simulink model "FCS_MPC_6ph_Regelungsmodell"  (R2022a)
settings: Solver=ode23t  StartTime=0.0  StopTime=0.1  RelTol=1e-3  AbsTol=1e-3  EnableMultiTasking=on
values from neighbouring files (symbols this model uses):
  f_c = 100000    [Params_testbench.m]
  L_d = 0.0001473    [Params_testbench.m]
  L_q = 0.0001484    [Params_testbench.m]
  L_x = 0.00005566    (= 5.566e-05)    [Params_testbench.m]
  L_y = L_x    (= 5.566e-05)    [Params_testbench.m]
  p = 5    [Params_testbench.m]
  psi_pm = 0.0048    [Params_testbench.m]
  R_ph = 0.1278    [Params_testbench.m]
  T_100MHz = 1/f_100MHz    (= 1e-08)    [Params_testbench.m]
  u_dc = 36.0    (= 36)    [Params_testbench.m]
libraries: hdlsllib x53, nesl_utility x39, fl_lib x32, ee_lib x12, simulink x8, spsAlphaBetaZerotodq0Lib x1
(part 6 of 8)

== system FCS_MPC_6ph_Regelungsmodell/Microcontroller Software/Prediction_and_cost_function1/Subsystem ==
  d_phase_voltage_per_switching_state : Inport
  q_phase_voltage_per_switching_state : Inport  Port=2
  x_phase_voltage_per_switching_state : Inport  Port=3
  y_phase_voltage_per_switching_state : Inport  Port=4
  d_phase_voltage_per_switching_state1 : Inport  Port=5
  q_phase_voltage_per_switching_state1 : Inport  Port=6
  x_phase_voltage_per_switching_state1 : Inport  Port=7
  y_phase_voltage_per_switching_state1 : Inport  Port=8
  d_phase_voltage_per_switching_state2 : Inport  Port=9
  q_phase_voltage_per_switching_state2 : Inport  Port=10
  x_phase_voltage_per_switching_state2 : Inport  Port=11
  y_phase_voltage_per_switching_state2 : Inport  Port=12
  d_phase_voltage_per_switching_state3 : Inport  Port=13
  q_phase_voltage_per_switching_state3 : Inport  Port=14
  x_phase_voltage_per_switching_state3 : Inport  Port=15
  y_phase_voltage_per_switching_state3 : Inport  Port=16
  d_phase_voltage_per_switching_state4 : Inport  Port=17
  q_phase_voltage_per_switching_state4 : Inport  Port=18
  x_phase_voltage_per_switching_state4 : Inport  Port=19
  y_phase_voltage_per_switching_state4 : Inport  Port=20
  d_phase_voltage_per_switching_state5 : Inport  Port=21
  q_phase_voltage_per_switching_state5 : Inport  Port=22
  x_phase_voltage_per_switching_state5 : Inport  Port=23
  y_phase_voltage_per_switching_state5 : Inport  Port=24
  d_phase_voltage_per_switching_state6 : Inport  Port=25
  q_phase_voltage_per_switching_state6 : Inport  Port=26
  x_phase_voltage_per_switching_state6 : Inport  Port=27
  y_phase_voltage_per_switching_state6 : Inport  Port=28
  d_phase_voltage_per_switching_state7 : Inport  Port=29
  q_phase_voltage_per_switching_state7 : Inport  Port=30
  x_phase_voltage_per_switching_state7 : Inport  Port=31
  y_phase_voltage_per_switching_state7 : Inport  Port=32
  SampleTime_div_Ld15 : Inport  Port=33
  SampleTime_div_Lq15 : Inport  Port=34
  SampleTime_div_Lx15 : Inport  Port=35
  SampleTime_div_Ly15 : Inport  Port=36
  id_k_16 : Inport  Port=37
  iq_k_16 : Inport  Port=38
  ix_k_16 : Inport  Port=39
  iy_k_16 : Inport  Port=40
  Rs15 : Inport  Port=41
  omega_el15 : Inport  Port=42
  Lq15 : Inport  Port=43
  Ld15 : Inport  Port=44
  psiPM15 : Inport  Port=45
  id_ref15 : Inport  Port=46
  iq_ref15 : Inport  Port=47
  ix_ref15 : Inport  Port=48
  iy_ref15 : Inport  Port=49
  MATLAB Function10 : MATLAB Function  TreatAsAtomicUnit=on
  MATLAB Function11 : MATLAB Function  TreatAsAtomicUnit=on
  MATLAB Function12 : MATLAB Function  TreatAsAtomicUnit=on
  MATLAB Function13 : MATLAB Function  TreatAsAtomicUnit=on
  MATLAB Function14 : MATLAB Function  TreatAsAtomicUnit=on
  MATLAB Function15 : MATLAB Function  TreatAsAtomicUnit=on
  MATLAB Function8 : MATLAB Function  TreatAsAtomicUnit=on
  MATLAB Function9 : MATLAB Function  TreatAsAtomicUnit=on
  J : Outport
  J1 : Outport  Port=2
  J2 : Outport  Port=3
  J3 : Outport  Port=4
  J4 : Outport  Port=5
  J5 : Outport  Port=6
  J6 : Outport  Port=7
  J7 : Outport  Port=8
  wires:
  q_phase_voltage_per_switching_state1/1 -> MATLAB Function14/15(q_phase_voltage_per_switching_state)
  SampleTime_div_Ld15/1 -> MATLAB Function8/1(SampleTime_div_Ld), MATLAB Function9/1(SampleTime_div_Ld), MATLAB Function10/1(SampleTime_div_Ld), MATLAB Function11/1(SampleTime_div_Ld), MATLAB Function12/1(SampleTime_div_Ld), MATLAB Function13/1(SampleTime_div_Ld), MATLAB Function14/1(SampleTime_div_Ld), MATLAB Function15/1(SampleTime_div_Ld)
  Rs15/1 -> MATLAB Function8/9(Rs), MATLAB Function9/9(Rs), MATLAB Function10/9(Rs), MATLAB Function11/9(Rs), MATLAB Function12/9(Rs), MATLAB Function13/9(Rs), MATLAB Function14/9(Rs), MATLAB Function15/9(Rs)
  y_phase_voltage_per_switching_state/1 -> MATLAB Function15/17(y_phase_voltage_per_switching_state)
  Lq15/1 -> MATLAB Function8/11(Lq), MATLAB Function9/11(Lq), MATLAB Function10/11(Lq), MATLAB Function11/11(Lq), MATLAB Function12/11(Lq), MATLAB Function13/11(Lq), MATLAB Function14/11(Lq), MATLAB Function15/11(Lq)
  MATLAB Function11/1(J) -> J4/1
  y_phase_voltage_per_switching_state2/1 -> MATLAB Function13/17(y_phase_voltage_per_switching_state)
  d_phase_voltage_per_switching_state1/1 -> MATLAB Function14/14(d_phase_voltage_per_switching_state)
  x_phase_voltage_per_switching_state1/1 -> MATLAB Function14/16(x_phase_voltage_per_switching_state)
  y_phase_voltage_per_switching_state7/1 -> MATLAB Function8/17(y_phase_voltage_per_switching_state)
  iy_ref15/1 -> MATLAB Function8/21(iy_ref), MATLAB Function9/21(iy_ref), MATLAB Function10/21(iy_ref), MATLAB Function11/21(iy_ref), MATLAB Function12/21(iy_ref), MATLAB Function13/21(iy_ref), MATLAB Function14/21(iy_ref), MATLAB Function15/21(iy_ref)
  omega_el15/1 -> MATLAB Function8/10(omega_el), MATLAB Function9/10(omega_el), MATLAB Function10/10(omega_el), MATLAB Function11/10(omega_el), MATLAB Function12/10(omega_el), MATLAB Function13/10(omega_el), MATLAB Function14/10(omega_el), MATLAB Function15/10(omega_el)
  psiPM15/1 -> MATLAB Function8/13(psiPM), MATLAB Function9/13(psiPM), MATLAB Function10/13(psiPM), MATLAB Function11/13(psiPM), MATLAB Function12/13(psiPM), MATLAB Function13/13(psiPM), MATLAB Function14/13(psiPM), MATLAB Function15/13(psiPM)
  d_phase_voltage_per_switching_state3/1 -> MATLAB Function12/14(d_phase_voltage_per_switching_state)
  d_phase_voltage_per_switching_state6/1 -> MATLAB Function9/14(d_phase_voltage_per_switching_state)
  d_phase_voltage_per_switching_state/1 -> MATLAB Function15/14(d_phase_voltage_per_switching_state)
  x_phase_voltage_per_switching_state3/1 -> MATLAB Function12/16(x_phase_voltage_per_switching_state)
  d_phase_voltage_per_switching_state2/1 -> MATLAB Function13/14(d_phase_voltage_per_switching_state)
  x_phase_voltage_per_switching_state4/1 -> MATLAB Function11/16(x_phase_voltage_per_switching_state)
  y_phase_voltage_per_switching_state1/1 -> MATLAB Function14/17(y_phase_voltage_per_switching_state)
  MATLAB Function14/1(J) -> J1/1
  MATLAB Function8/1(J) -> J7/1
  q_phase_voltage_per_switching_state2/1 -> MATLAB Function13/15(q_phase_voltage_per_switching_state)
  x_phase_voltage_per_switching_state2/1 -> MATLAB Function13/16(x_phase_voltage_per_switching_state)
  MATLAB Function13/1(J) -> J2/1
  y_phase_voltage_per_switching_state4/1 -> MATLAB Function11/17(y_phase_voltage_per_switching_state)
  x_phase_voltage_per_switching_state/1 -> MATLAB Function15/16(x_phase_voltage_per_switching_state)
  q_phase_voltage_per_switching_state5/1 -> MATLAB Function10/15(q_phase_voltage_per_switching_state)
  d_phase_voltage_per_switching_state7/1 -> MATLAB Function8/14(d_phase_voltage_per_switching_state)
  d_phase_voltage_per_switching_state4/1 -> MATLAB Function11/14(d_phase_voltage_per_switching_state)
  q_phase_voltage_per_switching_state4/1 -> MATLAB Function11/15(q_phase_voltage_per_switching_state)
  x_phase_voltage_per_switching_state5/1 -> MATLAB Function10/16(x_phase_voltage_per_switching_state)
  SampleTime_div_Lx15/1 -> MATLAB Function8/3(SampleTime_div_Lx), MATLAB Function9/3(SampleTime_div_Lx), MATLAB Function10/3(SampleTime_div_Lx), MATLAB Function11/3(SampleTime_div_Lx), MATLAB Function12/3(SampleTime_div_Lx), MATLAB Function13/3(SampleTime_div_Lx), MATLAB Function14/3(SampleTime_div_Lx), MATLAB Function15/3(SampleTime_div_Lx)
  SampleTime_div_Ly15/1 -> MATLAB Function8/4(SampleTime_div_Ly), MATLAB Function9/4(SampleTime_div_Ly), MATLAB Function10/4(SampleTime_div_Ly), MATLAB Function11/4(SampleTime_div_Ly), MATLAB Function12/4(SampleTime_div_Ly), MATLAB Function13/4(SampleTime_div_Ly), MATLAB Function14/4(SampleTime_div_Ly), MATLAB Function15/4(SampleTime_div_Ly)
  SampleTime_div_Lq15/1 -> MATLAB Function8/2(SampleTime_div_Lq), MATLAB Function9/2(SampleTime_div_Lq), MATLAB Function10/2(SampleTime_div_Lq), MATLAB Function11/2(SampleTime_div_Lq), MATLAB Function12/2(SampleTime_div_Lq), MATLAB Function13/2(SampleTime_div_Lq), MATLAB Function14/2(SampleTime_div_Lq), MATLAB Function15/2(SampleTime_div_Lq)
  x_phase_voltage_per_switching_state7/1 -> MATLAB Function8/16(x_phase_voltage_per_switching_state)
  q_phase_voltage_per_switching_state/1 -> MATLAB Function15/15(q_phase_voltage_per_switching_state)
  MATLAB Function15/1(J) -> J/1
  d_phase_voltage_per_switching_state5/1 -> MATLAB Function10/14(d_phase_voltage_per_switching_state)
  MATLAB Function10/1(J) -> J5/1
  y_phase_voltage_per_switching_state5/1 -> MATLAB Function10/17(y_phase_voltage_per_switching_state)
  q_phase_voltage_per_switching_state6/1 -> MATLAB Function9/15(q_phase_voltage_per_switching_state)
  y_phase_voltage_per_switching_state6/1 -> MATLAB Function9/17(y_phase_voltage_per_switching_state)
  x_phase_voltage_per_switching_state6/1 -> MATLAB Function9/16(x_phase_voltage_per_switching_state)
  MATLAB Function9/1(J) -> J6/1
  MATLAB Function12/1(J) -> J3/1
  q_phase_voltage_per_switching_state7/1 -> MATLAB Function8/15(q_phase_voltage_per_switching_state)
  y_phase_voltage_per_switching_state3/1 -> MATLAB Function12/17(y_phase_voltage_per_switching_state)
  q_phase_voltage_per_switching_state3/1 -> MATLAB Function12/15(q_phase_voltage_per_switching_state)
  ix_ref15/1 -> MATLAB Function8/20(ix_ref), MATLAB Function9/20(ix_ref), MATLAB Function10/20(ix_ref), MATLAB Function11/20(ix_ref), MATLAB Function12/20(ix_ref), MATLAB Function13/20(ix_ref), MATLAB Function14/20(ix_ref), MATLAB Function15/20(ix_ref)
  iq_ref15/1 -> MATLAB Function8/19(iq_ref), MATLAB Function9/19(iq_ref), MATLAB Function10/19(iq_ref), MATLAB Function11/19(iq_ref), MATLAB Function12/19(iq_ref), MATLAB Function13/19(iq_ref), MATLAB Function14/19(iq_ref), MATLAB Function15/19(iq_ref)
  id_ref15/1 -> MATLAB Function8/18(id_ref), MATLAB Function9/18(id_ref), MATLAB Function10/18(id_ref), MATLAB Function11/18(id_ref), MATLAB Function12/18(id_ref), MATLAB Function13/18(id_ref), MATLAB Function14/18(id_ref), MATLAB Function15/18(id_ref)
  Ld15/1 -> MATLAB Function8/12(Ld), MATLAB Function9/12(Ld), MATLAB Function10/12(Ld), MATLAB Function11/12(Ld), MATLAB Function12/12(Ld), MATLAB Function13/12(Ld), MATLAB Function14/12(Ld), MATLAB Function15/12(Ld)
  iy_k_16/1 -> MATLAB Function8/8(iy_k_1), MATLAB Function9/8(iy_k_1), MATLAB Function10/8(iy_k_1), MATLAB Function11/8(iy_k_1), MATLAB Function12/8(iy_k_1), MATLAB Function13/8(iy_k_1), MATLAB Function14/8(iy_k_1), MATLAB Function15/8(iy_k_1)
  ix_k_16/1 -> MATLAB Function8/7(ix_k_1), MATLAB Function9/7(ix_k_1), MATLAB Function10/7(ix_k_1), MATLAB Function11/7(ix_k_1), MATLAB Function12/7(ix_k_1), MATLAB Function13/7(ix_k_1), MATLAB Function14/7(ix_k_1), MATLAB Function15/7(ix_k_1)
  iq_k_16/1 -> MATLAB Function8/6(iq_k_1), MATLAB Function9/6(iq_k_1), MATLAB Function10/6(iq_k_1), MATLAB Function11/6(iq_k_1), MATLAB Function12/6(iq_k_1), MATLAB Function13/6(iq_k_1), MATLAB Function14/6(iq_k_1), MATLAB Function15/6(iq_k_1)
  id_k_16/1 -> MATLAB Function8/5(id_k_1), MATLAB Function9/5(id_k_1), MATLAB Function10/5(id_k_1), MATLAB Function11/5(id_k_1), MATLAB Function12/5(id_k_1), MATLAB Function13/5(id_k_1), MATLAB Function14/5(id_k_1), MATLAB Function15/5(id_k_1)

== matlab function FCS_MPC_6ph_Regelungsmodell/Microcontroller Software/Phase_voltages_per_switching_state2/MATLAB Function1 ==
  settings: fimath=fimath('RoundingMethod', 'Floor','OverflowAction', 'Wrap','ProductMode', 'FullPrecision', 'SumMode', 'FullPrecision')
  data: u input; y output
function y = fcn(u)

    y = fi(u*(1/(2*pi)));

end

== matlab function FCS_MPC_6ph_Regelungsmodell/Microcontroller Software/vsd_and_park_tra1/MATLAB Function ==
  settings: fimath=fimath('RoundingMethod', 'Floor','OverflowAction', 'Wrap','ProductMode', 'FullPrecision', 'SumMode', 'FullPrecision')
  data: i_a1 input; i_alpha output; i_b1 input; i_c1 input; i_a2 input; i_b2 input; i_c2 input; sin_theta_el input; i_beta output; i_x output; i_y output; i_0_plus output; i_0_minus output; i_d output; i_q output; cos_theta_el input
function [i_alpha,i_beta,i_x,i_y,i_0_plus,i_0_minus,i_d,i_q] = VSD_and_Park_transformation(i_a1,i_b1,i_c1,i_a2,i_b2,i_c2,sin_theta_el,cos_theta_el)

    % VSD-Transformation
    A = [0 0 0 0 0 0]';

    A =  0.3333*[1    -0.5        -0.5        0.8660   -0.8660  0 ;
                0    0.8660   -0.8660  0.5         0.5         -1;
                1    -0.5        -0.5        -0.8660  0.8660   0 ;
                0    -0.8660  0.8660   0.5         0.5         -1;
                1    1           1           0           0           0 ;
                0    0           0           1           1           1] * [i_a1 i_b1 i_c1 i_a2 i_b2 i_c2]';

    i_alpha = A(1);
    i_beta = A(2);
    i_x = A(3);
    i_y = A(4);
    i_0_plus = A(5);
    i_0_minus = A(6);

    % Park-Transformation
%    B = [0 0]';

%     B = [cos(theta_el)       sin(theta_el);
%         -sin(theta_el)       cos(theta_el)] * [i_alpha i_beta]';

 %   i_d = B(1);
 %   i_q = B(2);



i_d = cos_theta_el*i_alpha+sin_theta_el*i_beta;
i_q = -sin_theta_el*i_alpha+cos_theta_el*i_beta;


end

== matlab function FCS_MPC_6ph_Regelungsmodell/Microcontroller Software/vsd_and_park_tra1/MATLAB Function1 ==
  settings: fimath=fimath('RoundingMethod', 'Floor','OverflowAction', 'Wrap','ProductMode', 'FullPrecision', 'SumMode', 'FullPrecision')
  data: u input; y output
function y = fcn(u)

    y = u*(1/(2*pi));

end

== matlab function FCS_MPC_6ph_Regelungsmodell/Microcontroller Software/Delay_compensation1/MATLAB Function ==
  data: SampleTime_div_Ld input; SampleTime_div_Lq input; SampleTime_div_Lx input; SampleTime_div_Ly input; id_k_1 output; last_applied_optimal_voltage_d input; last_applied_optimal_voltage_q input; last_applied_optimal_voltage_x input; last_applied_optimal_voltage_y input; id_measured input; iq_measured input; ix_measured input; iy_measured input; psiPM input; Lq input; Ld input; Rs input; iq_k_1 output; ix_k_1 output; iy_k_1 output; omega_el input
function [id_k_1, iq_k_1, ix_k_1, iy_k_1] = fcn(SampleTime_div_Ld, SampleTime_div_Lq, SampleTime_div_Lx, SampleTime_div_Ly, last_applied_optimal_voltage_d, last_applied_optimal_voltage_q, last_applied_optimal_voltage_x, last_applied_optimal_voltage_y, id_measured, iq_measured, ix_measured, iy_measured, psiPM, Lq, Ld, Rs, omega_el)
  
    % Delay compensation with a modell of a 6-Phase PMSM
    id_k_1 = single(SampleTime_div_Ld*(last_applied_optimal_voltage_d-id_measured*Rs+omega_el*Lq*iq_measured)+id_measured);
    iq_k_1 = single(SampleTime_div_Lq*(last_applied_optimal_voltage_q-iq_measured*Rs-omega_el*(psiPM+id_measured*Ld))+iq_measured);
    ix_k_1 = single(SampleTime_div_Lx*(last_applied_optimal_voltage_x-ix_measured*Rs)+ix_measured);
    iy_k_1 = single(SampleTime_div_Ly*(last_applied_optimal_voltage_y-iy_measured*Rs)+iy_measured);

end

== matlab function FCS_MPC_6ph_Regelungsmodell/Microcontroller Software/Prediction_and_cost_function1/Subsystem/MATLAB Function10 ==
  data: SampleTime_div_Ld input; J output; SampleTime_div_Lq input; SampleTime_div_Lx input; SampleTime_div_Ly input; id_k_1 input; iq_k_1 input; ix_k_1 input; iy_k_1 input; Rs input; omega_el input; Lq input; Ld input; psiPM input; d_phase_voltage_per_switching_state input; q_phase_voltage_per_switching_state input; x_phase_voltage_per_switching_state input; y_phase_voltage_per_switching_state input; id_ref input; iq_ref input; ix_ref input; iy_ref input
function J = fcn(SampleTime_div_Ld, SampleTime_div_Lq, SampleTime_div_Lx, SampleTime_div_Ly, id_k_1, iq_k_1, ix_k_1, iy_k_1, Rs, omega_el, Lq, Ld, psiPM, d_phase_voltage_per_switching_state, q_phase_voltage_per_switching_state, x_phase_voltage_per_switching_state, y_phase_voltage_per_switching_state, id_ref, iq_ref, ix_ref, iy_ref)
     
        % Prediction of the d-, q-, x-, y-currents of the 6-Phase-PMSM with the finite control set 
        id_k_2 = single(SampleTime_div_Ld*(d_phase_voltage_per_switching_state-id_k_1*Rs+omega_el*Lq*iq_k_1)+id_k_1);
        iq_k_2 = single(SampleTime_div_Lq*(q_phase_voltage_per_switching_state-iq_k_1*Rs-omega_el*(psiPM+id_k_1*Ld))+iq_k_1);
        ix_k_2 = single(SampleTime_div_Lx*(x_phase_voltage_per_switching_state-ix_k_1*Rs)+ix_k_1);
        iy_k_2 = single(SampleTime_div_Ly*(y_phase_voltage_per_switching_state-iy_k_1*Rs)+iy_k_1);
        
        % Calculation of the cost function
        J = single((id_ref-id_k_2)^2+(iq_ref-iq_k_2)^2+(ix_ref-ix_k_2)^2+(iy_ref-iy_k_2)^2);

end

== matlab function FCS_MPC_6ph_Regelungsmodell/Microcontroller Software/Prediction_and_cost_function1/Subsystem/MATLAB Function11 ==
  data: SampleTime_div_Ld input; J output; SampleTime_div_Lq input; SampleTime_div_Lx input; SampleTime_div_Ly input; id_k_1 input; iq_k_1 input; ix_k_1 input; iy_k_1 input; Rs input; omega_el input; Lq input; Ld input; psiPM input; d_phase_voltage_per_switching_state input; q_phase_voltage_per_switching_state input; x_phase_voltage_per_switching_state input; y_phase_voltage_per_switching_state input; id_ref input; iq_ref input; ix_ref input; iy_ref input
function J = fcn(SampleTime_div_Ld, SampleTime_div_Lq, SampleTime_div_Lx, SampleTime_div_Ly, id_k_1, iq_k_1, ix_k_1, iy_k_1, Rs, omega_el, Lq, Ld, psiPM, d_phase_voltage_per_switching_state, q_phase_voltage_per_switching_state, x_phase_voltage_per_switching_state, y_phase_voltage_per_switching_state, id_ref, iq_ref, ix_ref, iy_ref)
     
        % Prediction of the d-, q-, x-, y-currents of the 6-Phase-PMSM with the finite control set 
        id_k_2 = single(SampleTime_div_Ld*(d_phase_voltage_per_switching_state-id_k_1*Rs+omega_el*Lq*iq_k_1)+id_k_1);
        iq_k_2 = single(SampleTime_div_Lq*(q_phase_voltage_per_switching_state-iq_k_1*Rs-omega_el*(psiPM+id_k_1*Ld))+iq_k_1);
        ix_k_2 = single(SampleTime_div_Lx*(x_phase_voltage_per_switching_state-ix_k_1*Rs)+ix_k_1);
        iy_k_2 = single(SampleTime_div_Ly*(y_phase_voltage_per_switching_state-iy_k_1*Rs)+iy_k_1);
        
        % Calculation of the cost function
        J = single((id_ref-id_k_2)^2+(iq_ref-iq_k_2)^2+(ix_ref-ix_k_2)^2+(iy_ref-iy_k_2)^2);

end

== matlab function FCS_MPC_6ph_Regelungsmodell/Microcontroller Software/Prediction_and_cost_function1/Subsystem/MATLAB Function12 ==
  data: SampleTime_div_Ld input; J output; SampleTime_div_Lq input; SampleTime_div_Lx input; SampleTime_div_Ly input; id_k_1 input; iq_k_1 input; ix_k_1 input; iy_k_1 input; Rs input; omega_el input; Lq input; Ld input; psiPM input; d_phase_voltage_per_switching_state input; q_phase_voltage_per_switching_state input; x_phase_voltage_per_switching_state input; y_phase_voltage_per_switching_state input; id_ref input; iq_ref input; ix_ref input; iy_ref input
function J = fcn(SampleTime_div_Ld, SampleTime_div_Lq, SampleTime_div_Lx, SampleTime_div_Ly, id_k_1, iq_k_1, ix_k_1, iy_k_1, Rs, omega_el, Lq, Ld, psiPM, d_phase_voltage_per_switching_state, q_phase_voltage_per_switching_state, x_phase_voltage_per_switching_state, y_phase_voltage_per_switching_state, id_ref, iq_ref, ix_ref, iy_ref)
     
        % Prediction of the d-, q-, x-, y-currents of the 6-Phase-PMSM with the finite control set 
        id_k_2 = single(SampleTime_div_Ld*(d_phase_voltage_per_switching_state-id_k_1*Rs+omega_el*Lq*iq_k_1)+id_k_1);
        iq_k_2 = single(SampleTime_div_Lq*(q_phase_voltage_per_switching_state-iq_k_1*Rs-omega_el*(psiPM+id_k_1*Ld))+iq_k_1);
        ix_k_2 = single(SampleTime_div_Lx*(x_phase_voltage_per_switching_state-ix_k_1*Rs)+ix_k_1);
        iy_k_2 = single(SampleTime_div_Ly*(y_phase_voltage_per_switching_state-iy_k_1*Rs)+iy_k_1);
        
        % Calculation of the cost function
        J = single((id_ref-id_k_2)^2+(iq_ref-iq_k_2)^2+(ix_ref-ix_k_2)^2+(iy_ref-iy_k_2)^2);

end

== matlab function FCS_MPC_6ph_Regelungsmodell/Microcontroller Software/Prediction_and_cost_function1/Subsystem/MATLAB Function13 ==
  data: SampleTime_div_Ld input; J output; SampleTime_div_Lq input; SampleTime_div_Lx input; SampleTime_div_Ly input; id_k_1 input; iq_k_1 input; ix_k_1 input; iy_k_1 input; Rs input; omega_el input; Lq input; Ld input; psiPM input; d_phase_voltage_per_switching_state input; q_phase_voltage_per_switching_state input; x_phase_voltage_per_switching_state input; y_phase_voltage_per_switching_state input; id_ref input; iq_ref input; ix_ref input; iy_ref input
function J = fcn(SampleTime_div_Ld, SampleTime_div_Lq, SampleTime_div_Lx, SampleTime_div_Ly, id_k_1, iq_k_1, ix_k_1, iy_k_1, Rs, omega_el, Lq, Ld, psiPM, d_phase_voltage_per_switching_state, q_phase_voltage_per_switching_state, x_phase_voltage_per_switching_state, y_phase_voltage_per_switching_state, id_ref, iq_ref, ix_ref, iy_ref)
     
        % Prediction of the d-, q-, x-, y-currents of the 6-Phase-PMSM with the finite control set 
        id_k_2 = single(SampleTime_div_Ld*(d_phase_voltage_per_switching_state-id_k_1*Rs+omega_el*Lq*iq_k_1)+id_k_1);
        iq_k_2 = single(SampleTime_div_Lq*(q_phase_voltage_per_switching_state-iq_k_1*Rs-omega_el*(psiPM+id_k_1*Ld))+iq_k_1);
        ix_k_2 = single(SampleTime_div_Lx*(x_phase_voltage_per_switching_state-ix_k_1*Rs)+ix_k_1);
        iy_k_2 = single(SampleTime_div_Ly*(y_phase_voltage_per_switching_state-iy_k_1*Rs)+iy_k_1);
        
        % Calculation of the cost function
        J = single((id_ref-id_k_2)^2+(iq_ref-iq_k_2)^2+(ix_ref-ix_k_2)^2+(iy_ref-iy_k_2)^2);

end

== matlab function FCS_MPC_6ph_Regelungsmodell/Microcontroller Software/Switching_states/MATLAB Function1 ==
  data: I input; next_switching_state output
function next_switching_state = fcn(I)

    % Possible switching states of the 6-Phase 2-level inverter
    possible_swichting_states = [0	1	0	1	0	1	0	1	0	1	0	1;
                                1	0	0	1	0	1	0	1	0	1	0	1;
                                0	1	1	0	0	1	0	1	0	1	0	1;
                                1	0	1	0	0	1	0	1	0	1	0	1;
                                0	1	0	1	1	0	0	1	0	1	0	1;
                                1	0	0	1	1	0	0	1	0	1	0	1;
                                0	1	1	0	1	0	0	1	0	1	0	1;
                                1	0	1	0	1	0	0	1	0	1	0	1;
                                0	1	0	1	0	1	1	0	0	1	0	1;
                                1	0	0	1	0	1	1	0	0	1	0	1;
                                0	1	1	0	0	1	1	0	0	1	0	1;
                                1	0	1	0	0	1	1	0	0	1	0	1;
                                0	1	0	1	1	0	1	0	0	1	0	1;
                                1	0	0	1	1	0	1	0	0	1	0	1;
                                0	1	1	0	1	0	1	0	0	1	0	1;
                                1	0	1	0	1	0	1	0	0	1	0	1;
                                0	1	0	1	0	1	0	1	1	0	0	1;
                                1	0	0	1	0	1	0	1	1	0	0	1;
                                0	1	1	0	0	1	0	1	1	0	0	1;
                                1	0	1	0	0	1	0	1	1	0	0	1;
                                0	1	0	1	1	0	0	1	1	0	0	1;
                                1	0	0	1	1	0	0	1	1	0	0	1;
                                0	1	1	0	1	0	0	1	1	0	0	1;
                                1	0	1	0	1	0	0	1	1	0	0	1;
                                0	1	0	1	0	1	1	0	1	0	0	1;
                                1	0	0	1	0	1	1	0	1	0	0	1;
                                0	1	1	0	0	1	1	0	1	0	0	1;
                                1	0	1	0	0	1	1	0	1	0	0	1;
                                0	1	0	1	1	0	1	0	1	0	0	1;
                                1	0	0	1	1	0	1	0	1	0	0	1;
                                0	1	1	0	1	0	1	0	1	0	0	1;
                                1	0	1	0	1	0	1	0	1	0	0	1;
                                0	1	0	1	0	1	0	1	0	1	1	0;
                                1	0	0	1	0	1	0	1	0	1	1	0;
                                0	1	1	0	0	1	0	1	0	1	1	0;
                                1	0	1	0	0	1	0	1	0	1	1	0;
                                0	1	0	1	1	0	0	1	0	1	1	0;
                                1	0	0	1	1	0	0	1	0	1	1	0;
                                0	1	1	0	1	0	0	1	0	1	1	0;
                                1	0	1	0	1	0	0	1	0	1	1	0;
                                0	1	0	1	0	1	1	0	0	1	1	0;
                                1	0	0	1	0	1	1	0	0	1	1	0;
                                0	1	1	0	0	1	1	0	0	1	1	0;
                                1	0	1	0	0	1	1	0	0	1	1	0;
                                0	1	0	1	1	0	1	0	0	1	1	0;
                                1	0	0	1	1	0	1	0	0	1	1	0;
                                0	1	1	0	1	0	1	0	0	1	1	0;
                                1	0	1	0	1	0	1	0	0	1	1	0;
                                0	1	0	1	0	1	0	1	1	0	1	0;
                                1	0	0	1	0	1	0	1	1	0	1	0;
                                0	1	1	0	0	1	0	1	1	0	1	0;
                                1	0	1	0	0	1	0	1	1	0	1	0;
                                0	1	0	1	1	0	0	1	1	0	1	0;
                                1	0	0	1	1	0	0	1	1	0	1	0;
                                0	1	1	0	1	0	0	1	1	0	1	0;
                                1	0	1	0	1	0	0	1	1	0	1	0;
                                0	1	0	1	0	1	1	0	1	0	1	0;
                                1	0	0	1	0	1	1	0	1	0	1	0;
                                0	1	1	0	0	1	1	0	1	0	1	0;
                                1	0	1	0	0	1	1	0	1	0	1	0;
                                0	1	0	1	1	0	1	0	1	0	1	0;
                                1	0	0	1	1	0	1	0	1	0	1	0;
                                0	1	1	0	1	0	1	0	1	0	1	0;
                                1	0	1	0	1	0	1	0	1	0	1	0];

    % Initial condition
    if I==0
        I=int32(1);
    end

    % Output switching state
    next_switching_state=boolean(possible_swichting_states(I,:))';

end

== matlab function FCS_MPC_6ph_Regelungsmodell/6ph_PMSM_30deg_VSD1 ==
  data: u1 input; y1 output; u2 input; u3 input; u4 input; u5 input; u6 input; y2 output; y3 output; y4 output; y5 output; y6 output; k6 input; c6 input
function [y1,y2,y3,y4,y5,y6] = VSD_asymm_30(u1,u2,u3,u4,u5,u6,k6,c6)

A =single([0 0 0 0 0 0]');

A =    k6*[1    -0.5        -0.5        sqrt(3)/2   -sqrt(3)/2  0 ;
           0    sqrt(3)/2   -sqrt(3)/2  0.5         0.5         -1;
           1    -0.5        -0.5        -sqrt(3)/2  sqrt(3)/2   0 ;
           0    -sqrt(3)/2  sqrt(3)/2   0.5         0.5         -1;
           c6   c6          c6          0           0           0 ;
           0    0           0           c6          c6          c6] * [u1 u2 u3 u4 u5 u6]';

y1 =single(A(1));
y2 =single(A(2));
y3 =single(A(3));
y4 =single(A(4));
y5 =single(A(5));
y6 =single(A(6));

== matlab function FCS_MPC_6ph_Regelungsmodell/Microcontroller Software/Prediction_and_cost_function1/Subsystem/MATLAB Function14 ==
  data: SampleTime_div_Ld input; J output; SampleTime_div_Lq input; SampleTime_div_Lx input; SampleTime_div_Ly input; id_k_1 input; iq_k_1 input; ix_k_1 input; iy_k_1 input; Rs input; omega_el input; Lq input; Ld input; psiPM input; d_phase_voltage_per_switching_state input; q_phase_voltage_per_switching_state input; x_phase_voltage_per_switching_state input; y_phase_voltage_per_switching_state input; id_ref input; iq_ref input; ix_ref input; iy_ref input
function J = fcn(SampleTime_div_Ld, SampleTime_div_Lq, SampleTime_div_Lx, SampleTime_div_Ly, id_k_1, iq_k_1, ix_k_1, iy_k_1, Rs, omega_el, Lq, Ld, psiPM, d_phase_voltage_per_switching_state, q_phase_voltage_per_switching_state, x_phase_voltage_per_switching_state, y_phase_voltage_per_switching_state, id_ref, iq_ref, ix_ref, iy_ref)
     
        % Prediction of the d-, q-, x-, y-currents of the 6-Phase-PMSM with the finite control set 
        id_k_2 = single(SampleTime_div_Ld*(d_phase_voltage_per_switching_state-id_k_1*Rs+omega_el*Lq*iq_k_1)+id_k_1);
        iq_k_2 = single(SampleTime_div_Lq*(q_phase_voltage_per_switching_state-iq_k_1*Rs-omega_el*(psiPM+id_k_1*Ld))+iq_k_1);
        ix_k_2 = single(SampleTime_div_Lx*(x_phase_voltage_per_switching_state-ix_k_1*Rs)+ix_k_1);
        iy_k_2 = single(SampleTime_div_Ly*(y_phase_voltage_per_switching_state-iy_k_1*Rs)+iy_k_1);
        
        % Calculation of the cost function
        J = single((id_ref-id_k_2)^2+(iq_ref-iq_k_2)^2+(ix_ref-ix_k_2)^2+(iy_ref-iy_k_2)^2);

end

== matlab function FCS_MPC_6ph_Regelungsmodell/Microcontroller Software/Prediction_and_cost_function1/Subsystem/MATLAB Function15 ==
  data: SampleTime_div_Ld input; J output; SampleTime_div_Lq input; SampleTime_div_Lx input; SampleTime_div_Ly input; id_k_1 input; iq_k_1 input; ix_k_1 input; iy_k_1 input; Rs input; omega_el input; Lq input; Ld input; psiPM input; d_phase_voltage_per_switching_state input; q_phase_voltage_per_switching_state input; x_phase_voltage_per_switching_state input; y_phase_voltage_per_switching_state input; id_ref input; iq_ref input; ix_ref input; iy_ref input
function J = fcn(SampleTime_div_Ld, SampleTime_div_Lq, SampleTime_div_Lx, SampleTime_div_Ly, id_k_1, iq_k_1, ix_k_1, iy_k_1, Rs, omega_el, Lq, Ld, psiPM, d_phase_voltage_per_switching_state, q_phase_voltage_per_switching_state, x_phase_voltage_per_switching_state, y_phase_voltage_per_switching_state, id_ref, iq_ref, ix_ref, iy_ref)
     
        % Prediction of the d-, q-, x-, y-currents of the 6-Phase-PMSM with the finite control set 
        id_k_2 = single(SampleTime_div_Ld*(d_phase_voltage_per_switching_state-id_k_1*Rs+omega_el*Lq*iq_k_1)+id_k_1);
        iq_k_2 = single(SampleTime_div_Lq*(q_phase_voltage_per_switching_state-iq_k_1*Rs-omega_el*(psiPM+id_k_1*Ld))+iq_k_1);
        ix_k_2 = single(SampleTime_div_Lx*(x_phase_voltage_per_switching_state-ix_k_1*Rs)+ix_k_1);
        iy_k_2 = single(SampleTime_div_Ly*(y_phase_voltage_per_switching_state-iy_k_1*Rs)+iy_k_1);
        
        % Calculation of the cost function
        J = single((id_ref-id_k_2)^2+(iq_ref-iq_k_2)^2+(ix_ref-ix_k_2)^2+(iy_ref-iy_k_2)^2);

end

== matlab function FCS_MPC_6ph_Regelungsmodell/Microcontroller Software/Prediction_and_cost_function1/Subsystem/MATLAB Function8 ==
  data: SampleTime_div_Ld input; J output; SampleTime_div_Lq input; SampleTime_div_Lx input; SampleTime_div_Ly input; id_k_1 input; iq_k_1 input; ix_k_1 input; iy_k_1 input; Rs input; omega_el input; Lq input; Ld input; psiPM input; d_phase_voltage_per_switching_state input; q_phase_voltage_per_switching_state input; x_phase_voltage_per_switching_state input; y_phase_voltage_per_switching_state input; id_ref input; iq_ref input; ix_ref input; iy_ref input
function J = fcn(SampleTime_div_Ld, SampleTime_div_Lq, SampleTime_div_Lx, SampleTime_div_Ly, id_k_1, iq_k_1, ix_k_1, iy_k_1, Rs, omega_el, Lq, Ld, psiPM, d_phase_voltage_per_switching_state, q_phase_voltage_per_switching_state, x_phase_voltage_per_switching_state, y_phase_voltage_per_switching_state, id_ref, iq_ref, ix_ref, iy_ref)
     
        % Prediction of the d-, q-, x-, y-currents of the 6-Phase-PMSM with the finite control set 
        id_k_2 = single(SampleTime_div_Ld*(d_phase_voltage_per_switching_state-id_k_1*Rs+omega_el*Lq*iq_k_1)+id_k_1);
        iq_k_2 = single(SampleTime_div_Lq*(q_phase_voltage_per_switching_state-iq_k_1*Rs-omega_el*(psiPM+id_k_1*Ld))+iq_k_1);
        ix_k_2 = single(SampleTime_div_Lx*(x_phase_voltage_per_switching_state-ix_k_1*Rs)+ix_k_1);
        iy_k_2 = single(SampleTime_div_Ly*(y_phase_voltage_per_switching_state-iy_k_1*Rs)+iy_k_1);
        
        % Calculation of the cost function
        J = single((id_ref-id_k_2)^2+(iq_ref-iq_k_2)^2+(ix_ref-ix_k_2)^2+(iy_ref-iy_k_2)^2);

end

== matlab function FCS_MPC_6ph_Regelungsmodell/Microcontroller Software/Prediction_and_cost_function1/Subsystem/MATLAB Function9 ==
  data: SampleTime_div_Ld input; J output; SampleTime_div_Lq input; SampleTime_div_Lx input; SampleTime_div_Ly input; id_k_1 input; iq_k_1 input; ix_k_1 input; iy_k_1 input; Rs input; omega_el input; Lq input; Ld input; psiPM input; d_phase_voltage_per_switching_state input; q_phase_voltage_per_switching_state input; x_phase_voltage_per_switching_state input; y_phase_voltage_per_switching_state input; id_ref input; iq_ref input; ix_ref input; iy_ref input
function J = fcn(SampleTime_div_Ld, SampleTime_div_Lq, SampleTime_div_Lx, SampleTime_div_Ly, id_k_1, iq_k_1, ix_k_1, iy_k_1, Rs, omega_el, Lq, Ld, psiPM, d_phase_voltage_per_switching_state, q_phase_voltage_per_switching_state, x_phase_voltage_per_switching_state, y_phase_voltage_per_switching_state, id_ref, iq_ref, ix_ref, iy_ref)
     
        % Prediction of the d-, q-, x-, y-currents of the 6-Phase-PMSM with the finite control set 
        id_k_2 = single(SampleTime_div_Ld*(d_phase_voltage_per_switching_state-id_k_1*Rs+omega_el*Lq*iq_k_1)+id_k_1);
        iq_k_2 = single(SampleTime_div_Lq*(q_phase_voltage_per_switching_state-iq_k_1*Rs-omega_el*(psiPM+id_k_1*Ld))+iq_k_1);
        ix_k_2 = single(SampleTime_div_Lx*(x_phase_voltage_per_switching_state-ix_k_1*Rs)+ix_k_1);
        iy_k_2 = single(SampleTime_div_Ly*(y_phase_voltage_per_switching_state-iy_k_1*Rs)+iy_k_1);
        
        % Calculation of the cost function
        J = single((id_ref-id_k_2)^2+(iq_ref-iq_k_2)^2+(ix_ref-ix_k_2)^2+(iy_ref-iy_k_2)^2);

end

== matlab function FCS_MPC_6ph_Regelungsmodell/Microcontroller Software/Min_cost_function_and_vopt1/MATLAB Function ==
  data: J_1 input fixdt(1,20,11); Index_1 input int32; J output fixdt(1,20,11); voltages_1 input fixdt(1,24,11); J_2 input fixdt(1,20,11); Index_2 input int32; voltages_2 input fixdt(1,24,11); J_3 input fixdt(1,20,11); Index_3 input int32; voltages_3 input fixdt(1,24,11); J_4 input fixdt(1,20,11); Index_4 input int32; voltages_4 input fixdt(1,24,11); J_5 input fixdt(1,20,11); Index_5 input int32; voltages_5 input fixdt(1,24,11); J_6 input fixdt(1,20,11); Index_6 input; voltages_6 input fixdt(1,24,11); J_7 input fixdt(1,20,11); Index_7 input int32; voltages_7 input fixdt(1,24,11); J_8 input fixdt(1,20,11); Index_8 input int32; voltages_8 input fixdt(1,24,11); Index output int32; voltages output fixdt(1,24,11); min input fixdt(1,20,11); J_default input fixdt(1,20,11); voltages_default input fixdt(1,24,11)
function [J, Index, voltages] = fcn(J_1, Index_1, voltages_1, J_2, Index_2, voltages_2, J_3, Index_3, voltages_3, J_4, Index_4, voltages_4, J_5, Index_5, voltages_5, J_6, Index_6, voltages_6, ...
                                    J_7, Index_7, voltages_7, J_8, Index_8, voltages_8, min, J_default,voltages_default)



if J_1 == min
    Index = Index_1;
    voltages = voltages_1;
    J = J_1;
elseif J_2 == min
    Index = Index_2;
    voltages = voltages_2;
    J = J_2;
elseif J_3 == min
    Index = Index_3;
    voltages = voltages_3;
    J = J_3;
elseif J_4 == min
    Index = Index_4;
    voltages = voltages_4;
    J = J_4;
elseif J_5 == min
    Index = Index_5;
    voltages = voltages_5;
    J = J_5;
elseif J_6 == min
    Index = Index_6;
    voltages = voltages_6;
    J = J_6;
elseif J_7 == min
    Index = Index_7;
    voltages = voltages_7;
    J = J_7;
elseif J_8 == min
    Index = Index_8;
    voltages = voltages_8;
    J = J_8;
else 
    Index = int32(0);
    J = J_default;
    voltages = voltages_default;
end

== matlab function FCS_MPC_6ph_Regelungsmodell/Microcontroller Software/Switching_states1/MATLAB Function1 ==
  data: I input; next_switching_state output
function next_switching_state = fcn(I)

    % Possible switching states of the 6-Phase 2-level inverter
    possible_swichting_states = [0	1	0	1	0	1	0	1	0	1	0	1;
                                1	0	0	1	0	1	0	1	0	1	0	1;
                                0	1	1	0	0	1	0	1	0	1	0	1;
                                1	0	1	0	0	1	0	1	0	1	0	1;
                                0	1	0	1	1	0	0	1	0	1	0	1;
                                1	0	0	1	1	0	0	1	0	1	0	1;
                                0	1	1	0	1	0	0	1	0	1	0	1;
                                1	0	1	0	1	0	0	1	0	1	0	1;
                                0	1	0	1	0	1	1	0	0	1	0	1;
                                1	0	0	1	0	1	1	0	0	1	0	1;
                                0	1	1	0	0	1	1	0	0	1	0	1;
                                1	0	1	0	0	1	1	0	0	1	0	1;
                                0	1	0	1	1	0	1	0	0	1	0	1;
                                1	0	0	1	1	0	1	0	0	1	0	1;
                                0	1	1	0	1	0	1	0	0	1	0	1;
                                1	0	1	0	1	0	1	0	0	1	0	1;
                                0	1	0	1	0	1	0	1	1	0	0	1;
                                1	0	0	1	0	1	0	1	1	0	0	1;
                                0	1	1	0	0	1	0	1	1	0	0	1;
                                1	0	1	0	0	1	0	1	1	0	0	1;
                                0	1	0	1	1	0	0	1	1	0	0	1;
                                1	0	0	1	1	0	0	1	1	0	0	1;
                                0	1	1	0	1	0	0	1	1	0	0	1;
                                1	0	1	0	1	0	0	1	1	0	0	1;
                                0	1	0	1	0	1	1	0	1	0	0	1;
                                1	0	0	1	0	1	1	0	1	0	0	1;
                                0	1	1	0	0	1	1	0	1	0	0	1;
                                1	0	1	0	0	1	1	0	1	0	0	1;
                                0	1	0	1	1	0	1	0	1	0	0	1;
                                1	0	0	1	1	0	1	0	1	0	0	1;
                                0	1	1	0	1	0	1	0	1	0	0	1;
                                1	0	1	0	1	0	1	0	1	0	0	1;
                                0	1	0	1	0	1	0	1	0	1	1	0;
                                1	0	0	1	0	1	0	1	0	1	1	0;
                                0	1	1	0	0	1	0	1	0	1	1	0;
                                1	0	1	0	0	1	0	1	0	1	1	0;
                                0	1	0	1	1	0	0	1	0	1	1	0;
                                1	0	0	1	1	0	0	1	0	1	1	0;
                                0	1	1	0	1	0	0	1	0	1	1	0;
                                1	0	1	0	1	0	0	1	0	1	1	0;
                                0	1	0	1	0	1	1	0	0	1	1	0;
                                1	0	0	1	0	1	1	0	0	1	1	0;
                                0	1	1	0	0	1	1	0	0	1	1	0;
                                1	0	1	0	0	1	1	0	0	1	1	0;
                                0	1	0	1	1	0	1	0	0	1	1	0;
                                1	0	0	1	1	0	1	0	0	1	1	0;
                                0	1	1	0	1	0	1	0	0	1	1	0;
                                1	0	1	0	1	0	1	0	0	1	1	0;
                                0	1	0	1	0	1	0	1	1	0	1	0;
                                1	0	0	1	0	1	0	1	1	0	1	0;
                                0	1	1	0	0	1	0	1	1	0	1	0;
                                1	0	1	0	0	1	0	1	1	0	1	0;
                                0	1	0	1	1	0	0	1	1	0	1	0;
                                1	0	0	1	1	0	0	1	1	0	1	0;
                                0	1	1	0	1	0	0	1	1	0	1	0;
                                1	0	1	0	1	0	0	1	1	0	1	0;
                                0	1	0	1	0	1	1	0	1	0	1	0;
                                1	0	0	1	0	1	1	0	1	0	1	0;
                                0	1	1	0	0	1	1	0	1	0	1	0;
                                1	0	1	0	0	1	1	0	1	0	1	0;
                                0	1	0	1	1	0	1	0	1	0	1	0;
                                1	0	0	1	1	0	1	0	1	0	1	0;
                                0	1	1	0	1	0	1	0	1	0	1	0;
                                1	0	1	0	1	0	1	0	1	0	1	0];

    % Initial condition
    if I==0
        I=int32(1);
    end

    % Output switching state
    next_switching_state=boolean(possible_swichting_states(I,:))';

end

== matlab function FCS_MPC_6ph_Regelungsmodell/Microcontroller Software/Phase_voltages_per_switching_state1/MATLAB Function1 ==
  settings: fimath=fimath('RoundingMethod', 'Floor','OverflowAction', 'Wrap','ProductMode', 'FullPrecision', 'SumMode', 'FullPrecision')
  data: u input; y output
function y = fcn(u)

    y = fi(u*(1/(2*pi)));

end

== matlab function FCS_MPC_6ph_Regelungsmodell/Microcontroller Software/Phase_voltages_per_switching_state1/Subsystem/MATLAB Function10 ==
  data: sin_theta_el input; cos_theta_el input; d_voltage_per_switching_state output; u_dc_link_voltage input; Index input; q_voltage_per_switching_state output; x_voltage_per_switching_state output; y_voltage_per_switching_state output
function [d_voltage_per_switching_state, q_voltage_per_switching_state, x_voltage_per_switching_state, y_voltage_per_switching_state] = fcn(sin_theta_el, cos_theta_el, u_dc_link_voltage, Index)
      
        % Initial condition
            Index = Index+1;

        % Swichtingstates factors alpha beta x y
        Factors_alpha_beta_x_y = single([0.288675134594813	 0.622008467928146	 0.122008467928146	 0.455341801261480    0.122008467928146	 0.455341801261480	-0.0446581987385205  0.288675134594813;
                                         -0.166666666666667	-0.166666666666667	 0.122008467928146	 0.122008467928146   -0.455341801261480	-0.455341801261480	-0.166666666666667	-0.166666666666667;
                                         -0.288675134594813	 0.0446581987385205	-0.455341801261480	-0.122008467928146   -0.455341801261480	-0.122008467928146	-0.622008467928146	-0.288675134594813;
                                         -0.166666666666667	-0.166666666666667	-0.455341801261480	-0.455341801261480    0.122008467928146	 0.122008467928146	-0.166666666666667	-0.166666666666667]);
        
        % Park-Transformation of the switchingstates factors
        Factors_d_q_x_y =single(zeros(4,1));
    
        Factors_d_q_x_y(3,1) = Factors_alpha_beta_x_y(3,Index);
        Factors_d_q_x_y(4,1) = Factors_alpha_beta_x_y(4,Index);
       
        Factors_d_q_x_y(1,1) = cos_theta_el*Factors_alpha_beta_x_y(1,Index)+sin_theta_el*Factors_alpha_beta_x_y(2,Index);
        Factors_d_q_x_y(2,1) = -sin_theta_el*Factors_alpha_beta_x_y(1,Index)+cos_theta_el*Factors_alpha_beta_x_y(2,Index);
    
        %Calculation of the voltages per switching state in alpha beta coordinates
        d_q_x_y_voltages_per_switching_state = single(u_dc_link_voltage*Factors_d_q_x_y);
    
        d_voltage_per_switching_state = d_q_x_y_voltages_per_switching_state(1,1);
        q_voltage_per_switching_state = d_q_x_y_voltages_per_switching_state(2,1);
        x_voltage_per_switching_state = d_q_x_y_voltages_per_switching_state(3,1);
        y_voltage_per_switching_state = d_q_x_y_voltages_per_switching_state(4,1);
    

end

== matlab function FCS_MPC_6ph_Regelungsmodell/Microcontroller Software/Phase_voltages_per_switching_state1/Subsystem/MATLAB Function11 ==
  data: sin_theta_el input; cos_theta_el input; d_voltage_per_switching_state output; u_dc_link_voltage input; Index input; q_voltage_per_switching_state output; x_voltage_per_switching_state output; y_voltage_per_switching_state output
function [d_voltage_per_switching_state, q_voltage_per_switching_state, x_voltage_per_switching_state, y_voltage_per_switching_state] = fcn(sin_theta_el, cos_theta_el, u_dc_link_voltage, Index)
      
        % Initial condition
            Index = Index+1;

    
        % Swichtingstates factors alpha beta x y
        Factors_alpha_beta_x_y = single([0	                 0.333333333333333	-0.166666666666667	  0.166666666666667    -0.166666666666667	  0.166666666666667	    -0.333333333333333	 0;
                                        -0.333333333333333	-0.333333333333333	-0.0446581987385205	 -0.0446581987385205   -0.622008467928146	 -0.622008467928146	    -0.333333333333333	-0.333333333333333;
                                         0	                 0.333333333333333	-0.166666666666667	  0.166666666666667    -0.166666666666667	  0.166666666666667	    -0.333333333333333	 0;
                                        -0.333333333333333	-0.333333333333333	-0.622008467928146	 -0.622008467928146    -0.0446581987385205   -0.0446581987385205	-0.333333333333333	-0.333333333333333]);
        
        % Park-Transformation of the switchingstates factors
        Factors_d_q_x_y =single(zeros(4,1));
    
        Factors_d_q_x_y(3,1) = Factors_alpha_beta_x_y(3,Index);
        Factors_d_q_x_y(4,1) = Factors_alpha_beta_x_y(4,Index);

        Factors_d_q_x_y(1,1) = cos_theta_el*Factors_alpha_beta_x_y(1,Index)+sin_theta_el*Factors_alpha_beta_x_y(2,Index);
        Factors_d_q_x_y(2,1) = -sin_theta_el*Factors_alpha_beta_x_y(1,Index)+cos_theta_el*Factors_alpha_beta_x_y(2,Index);
    
        %Calculation of the voltages per switching state in alpha beta coordinates
        d_q_x_y_voltages_per_switching_state = single(u_dc_link_voltage*Factors_d_q_x_y);
    
        d_voltage_per_switching_state = d_q_x_y_voltages_per_switching_state(1,1);
        q_voltage_per_switching_state = d_q_x_y_voltages_per_switching_state(2,1);
        x_voltage_per_switching_state = d_q_x_y_voltages_per_switching_state(3,1);
        y_voltage_per_switching_state = d_q_x_y_voltages_per_switching_state(4,1);
    

end

== matlab function FCS_MPC_6ph_Regelungsmodell/Microcontroller Software/Phase_voltages_per_switching_state1/Subsystem/MATLAB Function12 ==
  data: sin_theta_el input; cos_theta_el input; d_voltage_per_switching_state output; u_dc_link_voltage input; Index input; q_voltage_per_switching_state output; x_voltage_per_switching_state output; y_voltage_per_switching_state output
function [d_voltage_per_switching_state, q_voltage_per_switching_state, x_voltage_per_switching_state, y_voltage_per_switching_state] = fcn(sin_theta_el, cos_theta_el, u_dc_link_voltage, Index)
      
        % Initial condition
            Index = Index+1;

    
        % Swichtingstates factors alpha beta x y
        Factors_alpha_beta_x_y = single([0	                0.333333333333333	-0.166666666666667  	0.166666666666667   -0.166666666666667	 0.166666666666667	 -0.333333333333333	0;
                                         0.333333333333333	0.333333333333333	 0.622008467928146	    0.622008467928146    0.0446581987385205	 0.0446581987385205	  0.333333333333333	0.333333333333333;
                                         0	                0.333333333333333	-0.166666666666667	    0.166666666666667   -0.166666666666667	 0.166666666666667	 -0.333333333333333	0;
                                         0.333333333333333	0.333333333333333	 0.0446581987385205 	0.0446581987385205   0.622008467928146	 0.622008467928146	  0.333333333333333	0.333333333333333]);
        
        % Park-Transformation of the switchingstates factors
        Factors_d_q_x_y =single(zeros(4,1));
    
        Factors_d_q_x_y(3,1) = Factors_alpha_beta_x_y(3,Index);
        Factors_d_q_x_y(4,1) = Factors_alpha_beta_x_y(4,Index);
           
        Factors_d_q_x_y(1,1) = cos_theta_el*Factors_alpha_beta_x_y(1,Index)+sin_theta_el*Factors_alpha_beta_x_y(2,Index);
        Factors_d_q_x_y(2,1) = -sin_theta_el*Factors_alpha_beta_x_y(1,Index)+cos_theta_el*Factors_alpha_beta_x_y(2,Index);
    
        %Calculation of the voltages per switching state in alpha beta coordinates
        d_q_x_y_voltages_per_switching_state = single(u_dc_link_voltage*Factors_d_q_x_y);
    
        d_voltage_per_switching_state = d_q_x_y_voltages_per_switching_state(1,1);
        q_voltage_per_switching_state = d_q_x_y_voltages_per_switching_state(2,1);
        x_voltage_per_switching_state = d_q_x_y_voltages_per_switching_state(3,1);
        y_voltage_per_switching_state = d_q_x_y_voltages_per_switching_state(4,1);
    

end

== matlab function FCS_MPC_6ph_Regelungsmodell/Microcontroller Software/Phase_voltages_per_switching_state1/Subsystem/MATLAB Function13 ==
  data: sin_theta_el input; cos_theta_el input; d_voltage_per_switching_state output; u_dc_link_voltage input; Index input; q_voltage_per_switching_state output; x_voltage_per_switching_state output; y_voltage_per_switching_state output
function [d_voltage_per_switching_state, q_voltage_per_switching_state, x_voltage_per_switching_state, y_voltage_per_switching_state] = fcn(sin_theta_el, cos_theta_el, u_dc_link_voltage, Index)
      
        % Initial condition
            Index = Index+1;

    
        % Swichtingstates factors alpha beta x y
        Factors_alpha_beta_x_y = single([-0.288675134594813	0.0446581987385205	-0.455341801261480	-0.122008467928146   -0.455341801261480	-0.122008467928146	-0.622008467928146	-0.288675134594813;
                                         0.166666666666667	0.166666666666667	 0.455341801261480   0.455341801261480   -0.122008467928146	-0.122008467928146	 0.166666666666667	 0.166666666666667;
                                         0.288675134594813	0.622008467928146	 0.122008467928146	 0.455341801261480    0.122008467928146	 0.455341801261480	-0.0446581987385205	 0.288675134594813;
                                         0.166666666666667	0.166666666666667	-0.122008467928146	-0.122008467928146    0.455341801261480	 0.455341801261480	 0.166666666666667	 0.166666666666667]);
        
        % Park-Transformation of the switchingstates factors
        Factors_d_q_x_y =single(zeros(4,1));
    
        Factors_d_q_x_y(3,1) = Factors_alpha_beta_x_y(3,Index);
        Factors_d_q_x_y(4,1) = Factors_alpha_beta_x_y(4,Index);
           
        Factors_d_q_x_y(1,1) = cos_theta_el*Factors_alpha_beta_x_y(1,Index)+sin_theta_el*Factors_alpha_beta_x_y(2,Index);
        Factors_d_q_x_y(2,1) = -sin_theta_el*Factors_alpha_beta_x_y(1,Index)+cos_theta_el*Factors_alpha_beta_x_y(2,Index);
    
        %Calculation of the voltages per switching state in alpha beta coordinates
        d_q_x_y_voltages_per_switching_state = single(u_dc_link_voltage*Factors_d_q_x_y);
    
        d_voltage_per_switching_state = d_q_x_y_voltages_per_switching_state(1,1);
        q_voltage_per_switching_state = d_q_x_y_voltages_per_switching_state(2,1);
        x_voltage_per_switching_state = d_q_x_y_voltages_per_switching_state(3,1);
        y_voltage_per_switching_state = d_q_x_y_voltages_per_switching_state(4,1);
    

end
